simulink model "GalvoModel_v3_blockumbau"  (R2013a)
settings: Solver=ode45  StartTime=0.0  StopTime=20e-3  MaxStep=1e-6  RelTol=1e-3
undefined symbols (not defined in the file or in its folder): BEM, CL, CR, FR, KTR, RIN, TRC
libraries: simulink x2
settings Model: Creator=mainster  LastModifiedBy=mainster
settings DebuggingCC: SolverPrmCheckMsg=none

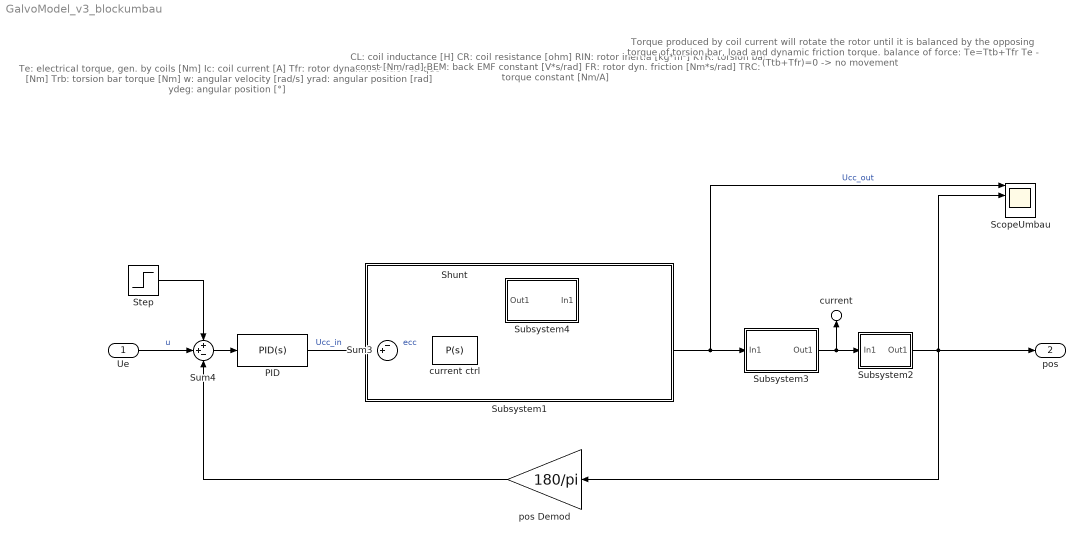
== system GalvoModel_v3_blockumbau ==
  note: Te: 	electrical torque, gen. by coils	[Nm]
      |  Ic: 	coil current							[A]
      |  Tfr:	rotor dynamic friction torque 		[Nm]
      |  Trb:	torsion bar torque					[Nm]
      |  w:		angular velocity 					[rad/s]
      |  yrad:	angular position 					[rad]
      |  ydeg:	angular position 					[°]
  note: CL:	coil inductance 		[H]
      |  CR:	coil resistance 		[ohm]
      |  RIN:	rotor inertia 			[kg*m²]
      |  KTR:	torsion bar const 	[Nm/rad]
      |  BEM:	back EMF constant	[V*s/rad]
      |  FR:	rotor dyn. friction	[Nm*s/rad]
      |  TRC:	torque constant		[Nm/A]
  note: Torque produced by coil current will rotate the rotor until
      | it is balanced by the opposing torque of torsion bar, load
      | and dynamic friction torque.
      | balance of force: 	Te=Ttb+Tfr
      | 						Te - (Ttb+Tfr)=0  ->  no movement
  Ue : Inport
  PID : simulink/Continuous/PID Controller  Controller=PID  TimeDomain=Continuous-time  SampleTime=1  IntegratorMethod=Forward Euler  FilterMethod=Forward Euler  Form=Parallel  P=0.118803398901385  I=41.4515194383798  D=8.41592067923308e-05  N=758717.459878032  InitialConditionSource=internal  InitialConditionForIntegrator=0  InitialConditionForFilter=0  ExternalReset=none  LimitOutput=on  UpperSaturationLimit=10  LowerSaturationLimit=-10  LinearizeAsGain=off  AntiWindupMode=none  Kb=1  TrackingMode=off  Kt=0  PParamMin=[]  PParamMax=[]  IParamMin=[]  IParamMax=[]  DParamMin=[]  DParamMax=[]  NParamMin=[]  NParamMax=[]  KbParamMin=[]  KbParamMax=[]  KtParamMin=[]  KtParamMax=[]  POutMin=[]  POutMax=[]  IOutMin=[]  IOutMax=[]  DOutMin=[]  DOutMax=[]  NOutMin=[]  NOutMax=[]  KbOutMin=[]  KbOutMax=[]  KtOutMin=[]  KtOutMax=[]  IntegratorOutMin=[]  IntegratorOutMax=[]  FilterOutMin=[]  FilterOutMax=[]  SumOutMin=[]  SumOutMax=[]  SumI1OutMin=[]  SumI1OutMax=[]  SumI2OutMin=[]  SumI2OutMax=[]  SumI3OutMin=[]  SumI3OutMax=[]  SumDOutMin=[]  SumDOutMax=[]  SaturationOutMin=[]  SaturationOutMax=[]  IntegratorContinuousStateAttributes=''  IntegratorStateMustResolveToSignalObject=off  IntegratorRTWStateStorageClass=Auto  FilterContinuousStateAttributes=''  FilterStateMustResolveToSignalObject=off  FilterRTWStateStorageClass=Auto
  ScopeUmbau : Scope  NumInputPorts=4
      settings: ShowLegends=on  TimeRange=0.02  YMin=-20~0~-1~-1  YMax=100~0.04~1~1  MaxDataPoints=500000
  Shunt : Gain  Gain=0.1
  Step : Step  Time=1e-3  After=2  SampleTime=0
      settings: AttributesFormatString=Ampl.: %<After>
  Subsystem1 : Subsystem  mask{d=0}
      mask Display: disp('')
  Subsystem2 : Subsystem
  Subsystem3 : Subsystem
  Subsystem4 : Subsystem
  Sum3 : Sum  Inputs=-+|
  Sum4 : Sum  Inputs=++-
  current ctrl : simulink/Continuous/PID Controller  Controller=P  TimeDomain=Continuous-time  SampleTime=1  IntegratorMethod=Forward Euler  FilterMethod=Forward Euler  Form=Parallel  P=10  I=0.7525  D=0.156  N=100  InitialConditionSource=internal  InitialConditionForIntegrator=0  InitialConditionForFilter=0  ExternalReset=none  LimitOutput=off  UpperSaturationLimit=10  LowerSaturationLimit=-10  LinearizeAsGain=off  AntiWindupMode=none  Kb=1  TrackingMode=off  Kt=1  PParamMin=[]  PParamMax=[]  IParamMin=[]  IParamMax=[]  DParamMin=[]  DParamMax=[]  NParamMin=[]  NParamMax=[]  KbParamMin=[]  KbParamMax=[]  KtParamMin=[]  KtParamMax=[]  POutMin=[]  POutMax=[]  IOutMin=[]  IOutMax=[]  DOutMin=[]  DOutMax=[]  NOutMin=[]  NOutMax=[]  KbOutMin=[]  KbOutMax=[]  KtOutMin=[]  KtOutMax=[]  IntegratorOutMin=[]  IntegratorOutMax=[]  FilterOutMin=[]  FilterOutMax=[]  SumOutMin=[]  SumOutMax=[]  SumI1OutMin=[]  SumI1OutMax=[]  SumI2OutMin=[]  SumI2OutMax=[]  SumI3OutMin=[]  SumI3OutMax=[]  SumDOutMin=[]  SumDOutMax=[]  SaturationOutMin=[]  SaturationOutMax=[]  IntegratorContinuousStateAttributes=''  IntegratorStateMustResolveToSignalObject=off  IntegratorRTWStateStorageClass=Auto  FilterContinuousStateAttributes=''  FilterStateMustResolveToSignalObject=off  FilterRTWStateStorageClass=Auto
  pos Demod : Gain  Gain=180/pi
  current : Outport
  pos : Outport  Port=2
  wires:
  Sum3/1 -> current ctrl/1  "ecc"
  Shunt/1 -> Sum3/1
  PID/1 -> Sum3/2  "Ucc_in"
  Sum4/1 -> PID/1
  current ctrl/1 -> Subsystem4/1(In1), ScopeUmbau/1, Subsystem3/1(In1)  "Ucc_out"
  Step/1 -> Sum4/1
  Ue/1 -> Sum4/2  "u"
  pos Demod/1 -> Sum4/3
  Subsystem3/1(Out1) -> Subsystem2/1(In1), current/1
  Subsystem4/1(Out1) -> Shunt/1
  Subsystem2/1(Out1) -> pos Demod/1, ScopeUmbau/2, pos/1

== system GalvoModel_v3_blockumbau/Subsystem1 ==

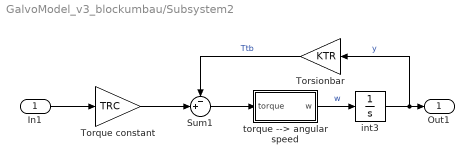
== system GalvoModel_v3_blockumbau/Subsystem2 ==
  In1 : Inport
  Sum1 : Sum  Inputs=-+|
  Torque constant : Gain  Gain=TRC
  Torsionbar : Gain  Gain=KTR
  int3 : Integrator
  torque --> angular speed : Subsystem
  Out1 : Outport
  wires:
  In1/1 -> Torque constant/1
  int3/1 -> Torsionbar/1, Out1/1  "y"
  Torsionbar/1 -> Sum1/1  "Ttb"
  torque --> angular speed/1(w) -> int3/1  "w"
  Sum1/1 -> torque --> angular speed/1(torque)
  Torque constant/1 -> Sum1/2

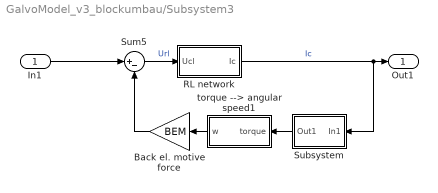
== system GalvoModel_v3_blockumbau/Subsystem3 ==
  In1 : Inport
  Back el. motive force : Gain  Gain=BEM
  RL network : Subsystem
  Subsystem : Subsystem
  Sum5 : Sum  Inputs=|+-
  torque --> angular speed1 : Subsystem
  Out1 : Outport
  wires:
  torque --> angular speed1/1(w) -> Back el. motive force/1
  In1/1 -> Sum5/1
  Subsystem/1(Out1) -> torque --> angular speed1/1(torque)
  Back el. motive force/1 -> Sum5/2
  Sum5/1 -> RL network/1(Ucl)  "Url"
  RL network/1(Ic) -> Subsystem/1(In1), Out1/1  "Ic"

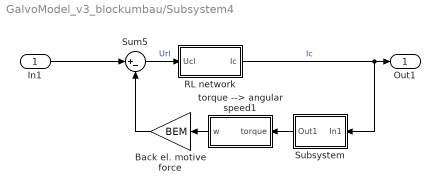
== system GalvoModel_v3_blockumbau/Subsystem4 ==
  In1 : Inport
  Back el. motive force : Gain  Gain=BEM
  RL network : Subsystem
  Subsystem : Subsystem
  Sum5 : Sum  Inputs=|+-
  torque --> angular speed1 : Subsystem
  Out1 : Outport
  wires:
  torque --> angular speed1/1(w) -> Back el. motive force/1
  In1/1 -> Sum5/1
  Subsystem/1(Out1) -> torque --> angular speed1/1(torque)
  Back el. motive force/1 -> Sum5/2
  Sum5/1 -> RL network/1(Ucl)  "Url"
  RL network/1(Ic) -> Subsystem/1(In1), Out1/1  "Ic"

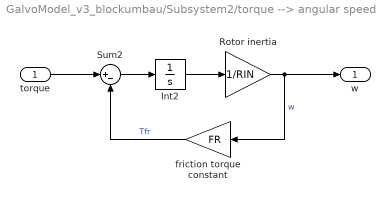
== system GalvoModel_v3_blockumbau/Subsystem2/torque --> angular speed ==
  torque : Inport
  Int2 : Integrator
  Rotor inertia : Gain  Gain=1/RIN
  Sum2 : Sum  Inputs=|+-
  friction torque constant : Gain  Gain=FR
  w : Outport
  wires:
  Int2/1 -> Rotor inertia/1
  Sum2/1 -> Int2/1
  Rotor inertia/1 -> w/1, friction torque constant/1  "w"
  torque/1 -> Sum2/1
  friction torque constant/1 -> Sum2/2  "Tfr"

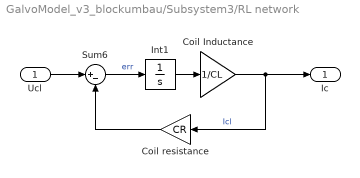
== system GalvoModel_v3_blockumbau/Subsystem3/RL network ==
  Ucl : Inport
  Coil Inductance : Gain  Gain=1/CL
  Coil resistance : Gain  Gain=CR
  Int1 : Integrator
  Sum6 : Sum  Inputs=|+-
      settings: AttributesFormatString=%<Name>
  Ic : Outport
  wires:
  Int1/1 -> Coil Inductance/1
  Coil resistance/1 -> Sum6/2
  Coil Inductance/1 -> Ic/1, Coil resistance/1  "Icl"
  Ucl/1 -> Sum6/1
  Sum6/1 -> Int1/1  "err"

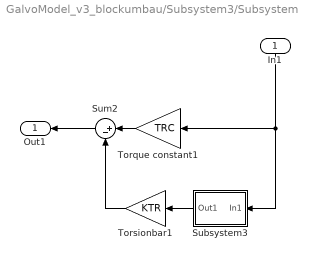
== system GalvoModel_v3_blockumbau/Subsystem3/Subsystem ==
  In1 : Inport
  Subsystem3 : Subsystem
  Sum2 : Sum  Inputs=|+-
  Torque constant1 : Gain  Gain=TRC
  Torsionbar1 : Gain  Gain=KTR
  Out1 : Outport
  wires:
  Subsystem3/1(Out1) -> Torsionbar1/1
  Torsionbar1/1 -> Sum2/2
  Sum2/1 -> Out1/1
  In1/1 -> Subsystem3/1(In1), Torque constant1/1
  Torque constant1/1 -> Sum2/1

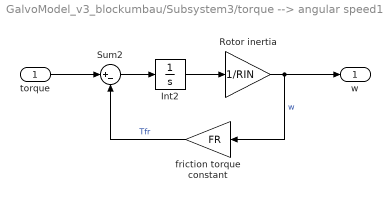
== system GalvoModel_v3_blockumbau/Subsystem3/torque --> angular speed1 ==
  torque : Inport
  Int2 : Integrator
  Rotor inertia : Gain  Gain=1/RIN
  Sum2 : Sum  Inputs=|+-
  friction torque constant : Gain  Gain=FR
  w : Outport
  wires:
  Int2/1 -> Rotor inertia/1
  Sum2/1 -> Int2/1
  Rotor inertia/1 -> w/1, friction torque constant/1  "w"
  torque/1 -> Sum2/1
  friction torque constant/1 -> Sum2/2  "Tfr"

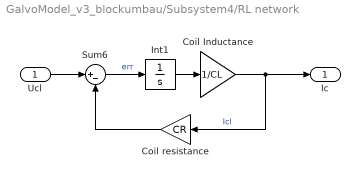
== system GalvoModel_v3_blockumbau/Subsystem4/RL network ==
  Ucl : Inport
  Coil Inductance : Gain  Gain=1/CL
  Coil resistance : Gain  Gain=CR
  Int1 : Integrator
  Sum6 : Sum  Inputs=|+-
      settings: AttributesFormatString=%<Name>
  Ic : Outport
  wires:
  Int1/1 -> Coil Inductance/1
  Coil resistance/1 -> Sum6/2
  Coil Inductance/1 -> Ic/1, Coil resistance/1  "Icl"
  Ucl/1 -> Sum6/1
  Sum6/1 -> Int1/1  "err"

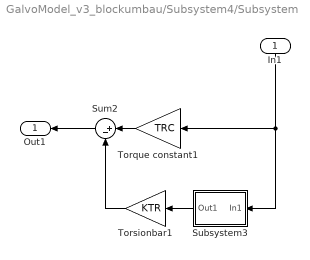
== system GalvoModel_v3_blockumbau/Subsystem4/Subsystem ==
  In1 : Inport
  Subsystem3 : Subsystem
  Sum2 : Sum  Inputs=|+-
  Torque constant1 : Gain  Gain=TRC
  Torsionbar1 : Gain  Gain=KTR
  Out1 : Outport
  wires:
  Subsystem3/1(Out1) -> Torsionbar1/1
  Torsionbar1/1 -> Sum2/2
  Sum2/1 -> Out1/1
  In1/1 -> Subsystem3/1(In1), Torque constant1/1
  Torque constant1/1 -> Sum2/1

== system GalvoModel_v3_blockumbau/Subsystem4/torque --> angular speed1 ==
  torque : Inport
  Int2 : Integrator
  Rotor inertia : Gain  Gain=1/RIN
  Sum2 : Sum  Inputs=|+-
  friction torque constant : Gain  Gain=FR
  w : Outport
  wires:
  Int2/1 -> Rotor inertia/1
  Sum2/1 -> Int2/1
  Rotor inertia/1 -> w/1, friction torque constant/1  "w"
  torque/1 -> Sum2/1
  friction torque constant/1 -> Sum2/2  "Tfr"

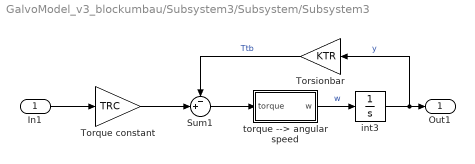
== system GalvoModel_v3_blockumbau/Subsystem3/Subsystem/Subsystem3 ==
  In1 : Inport
  Sum1 : Sum  Inputs=-+|
  Torque constant : Gain  Gain=TRC
  Torsionbar : Gain  Gain=KTR
  int3 : Integrator
  torque --> angular speed : Subsystem
  Out1 : Outport
  wires:
  In1/1 -> Torque constant/1
  int3/1 -> Torsionbar/1, Out1/1  "y"
  Torsionbar/1 -> Sum1/1  "Ttb"
  torque --> angular speed/1(w) -> int3/1  "w"
  Sum1/1 -> torque --> angular speed/1(torque)
  Torque constant/1 -> Sum1/2

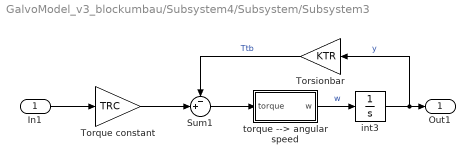
== system GalvoModel_v3_blockumbau/Subsystem4/Subsystem/Subsystem3 ==
  In1 : Inport
  Sum1 : Sum  Inputs=-+|
  Torque constant : Gain  Gain=TRC
  Torsionbar : Gain  Gain=KTR
  int3 : Integrator
  torque --> angular speed : Subsystem
  Out1 : Outport
  wires:
  In1/1 -> Torque constant/1
  int3/1 -> Torsionbar/1, Out1/1  "y"
  Torsionbar/1 -> Sum1/1  "Ttb"
  torque --> angular speed/1(w) -> int3/1  "w"
  Sum1/1 -> torque --> angular speed/1(torque)
  Torque constant/1 -> Sum1/2

== system GalvoModel_v3_blockumbau/Subsystem3/Subsystem/Subsystem3/torque --> angular speed ==
  torque : Inport
  Int2 : Integrator
  Rotor inertia : Gain  Gain=1/RIN
  Sum2 : Sum  Inputs=|+-
  friction torque constant : Gain  Gain=FR
  w : Outport
  wires:
  Int2/1 -> Rotor inertia/1
  Sum2/1 -> Int2/1
  Rotor inertia/1 -> w/1, friction torque constant/1  "w"
  torque/1 -> Sum2/1
  friction torque constant/1 -> Sum2/2  "Tfr"

== system GalvoModel_v3_blockumbau/Subsystem4/Subsystem/Subsystem3/torque --> angular speed ==
  torque : Inport
  Int2 : Integrator
  Rotor inertia : Gain  Gain=1/RIN
  Sum2 : Sum  Inputs=|+-
  friction torque constant : Gain  Gain=FR
  w : Outport
  wires:
  Int2/1 -> Rotor inertia/1
  Sum2/1 -> Int2/1
  Rotor inertia/1 -> w/1, friction torque constant/1  "w"
  torque/1 -> Sum2/1
  friction torque constant/1 -> Sum2/2  "Tfr"
